simulink model "heaveCompMichael_v04"  (R2022b)
settings: Solver=VariableStepAuto  StartTime=0.0  StopTime=20  RelTol=1e-3
model workspace (MATLAB code in the model file):
  | %fluid data
  | rho = 875;
  | %valve config
  | P_r = 70e5;
  | Cd = 0.7;
  | Q_r = 200/6e4;
  | AdMax = Q_r/Cd/sqrt(2/rho*P_r/2);
  | 
  | g = 9.81;                   %gravity
  | zw = 0.8;                   %wave amplitude
  | tw = 10;                    %total wave period
  | ig = 46;                    %gear ratio gearbox
  | m = 9000;                   %mass of payload
  | mueq = 0.15;                %friction coeffisient
  | dd = 0.45;                  %diameter drum
  | nyv = 0.92;                 %volumetric effissiency
  | rd = dd/2;                  %radius drum
  | omega0 = 5;                 %velosity in friction equation
  | omegap = 1500;              %velosity hpu pump
  | nsh = 3;
  | gearrationsh = nsh.*2;
libraries: fl_lib x40, nesl_utility x24, sh_lib x7, slpidlib x2
(part 2 of 2)

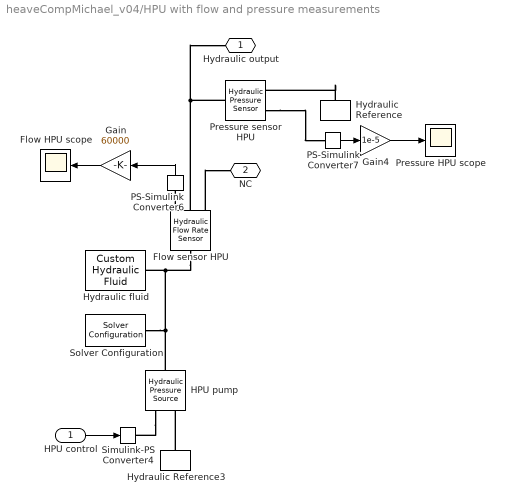
== system heaveCompMichael_v04/HPU with flow and pressure measurements ==
  HPU control : Inport
  Flow HPU scope : Scope
  Flow sensor HPU : fl_lib/Hydraulic/Hydraulic Sensors/Hydraulic Flow Rate Sensor
  Gain : Gain  Gain=60000
  Gain4 : Gain  Gain=1e-5
  HPU pump : fl_lib/Hydraulic/Hydraulic Sources/Hydraulic Pressure Source
      settings: InternalSimscapePortConfiguration="{\"Bottom\":[],\"Left\":[{\"id\":\"P\",\"label\":\"P\",\"type\":\"foundation.hydraulic.hydraulic\"}],\"Right\":[{\"id\":\"S\",\"label\":\"S\",\"type\":\"input\"},{\"id\":\"T\",\"label\":\"T\",\"type\":\"foundation.hydraulic.hydraulic\"}],\"Top\":[]}"
  Hydraulic Reference : fl_lib/Hydraulic/Hydraulic Elements/Hydraulic Reference
  Hydraulic Reference3 : fl_lib/Hydraulic/Hydraulic Elements/Hydraulic Reference
  Hydraulic fluid : fl_lib/Hydraulic/Hydraulic Utilities/Custom Hydraulic Fluid  density=875 kg/m^3  viscosity_kin=18e-6 m^2/s  bulk=0.8e9 Pa  alpha=0.005  range_error=2
      settings: InternalSimscapePortConfiguration="{\"Bottom\":[],\"Left\":[],\"Right\":[{\"id\":\"G\",\"label\":\"\",\"type\":\"foundation.hydraulic.hydraulic\"}],\"Top\":[]}"
  PS-Simulink Converter6 : nesl_utility/PS-Simulink Converter  PhysicalDomain=network_engine_domain  SubClassName=ps_output  LeftPortType=input  RightPortType=output  PseudoPeriodic=off  Frequencies=[]  VectorFormat=inherit  Unit=inherit  AffineConversion=off
  PS-Simulink Converter7 : nesl_utility/PS-Simulink Converter  PhysicalDomain=network_engine_domain  SubClassName=ps_output  LeftPortType=input  RightPortType=output  PseudoPeriodic=off  Frequencies=[]  VectorFormat=inherit  Unit=inherit  AffineConversion=off
  Pressure HPU scope : Scope
  Pressure sensor HPU : fl_lib/Hydraulic/Hydraulic Sensors/Hydraulic Pressure Sensor
  Simulink-PS Converter4 : nesl_utility/Simulink-PS Converter  PhysicalDomain=network_engine_domain  SubClassName=ps_input  LeftPortType=input  RightPortType=output  PseudoPeriodic=off  Frequencies=[]  NoiseDistribution=none  NoiseParameters=[]  Unit=1  AffineConversion=off  FilteringAndDerivatives=provide  SimscapeFilterOrder=1  InputFilterTimeConstant=0.001  UdotUserProvided=0
  Solver Configuration : nesl_utility/Solver Configuration  PhysicalDomain=network_engine_domain  SubClassName=solver  LeftPortType=input  RightPortType=generic  Tones=[]  Harmonics=[]  SimulateNoise=off  Profile=off  UseLocalSampling=off  EnableSwitchedLinearOptims=on  FrequencyDomain=off  UseCCode=off  RelTol=0.001  AbsTol=1e-06  MinStep=1e-09  ToWorkspace=off  RevertToSquareIcSolve=off  NumHomotopyIterations=100  PhasorMode=off  PhasorModeNumHarmonics=1  ConsistencySolver=NEWTON_FTOL  IndexReductionMethod=DerivativeReplacement  DoDC=off  ResidualTolerance=1e-09  ConsistencyTolSource=GLOBAL  ConsistencyAbsTol=0.001  ConsistencyRelTol=0.001  ConsistencyTolFactor=0.001  UseLocalSolver=off  LocalSolverChoice=NE_BACKWARD_EULER_ADVANCER  ResolveIndetEquations=on  FunctionEvalNumThread=1  LocalSolverSampleTime=0.001  DoFixedCost=off  MaxNonlinIter=3  MaxModeIter=2  ComputeImpulses=off  ImpulseIterations=2  LinearAlgebra=auto  LinearAlgebraNumThread=0  EquationFormulation=NE_TIME_EF  DelaysMemoryBudget=1024  AutomaticFiltering=on  FilteringTimeConstant=0.001  PartitionStorageMethod=AS_NEEDED  PartitionMemoryBudget=1024  PartitionMethod=ROBUST
  Hydraulic output : PMIOPort  Side=Right
  NC : PMIOPort  Port=2  Side=Right
  wires:
  PS-Simulink Converter6/1 -> Gain/1
  PS-Simulink Converter7/1 -> Gain4/1
  HPU control/1 -> Simulink-PS Converter4/1
  Gain/1 -> Flow HPU scope/1
  Gain4/1 -> Pressure HPU scope/1
  connections:
  HPU pump/LConn1 -- Solver Configuration/RConn1 -- Flow sensor HPU/LConn1 -- Hydraulic fluid/RConn1
  Hydraulic Reference3/LConn1 -- HPU pump/RConn2
  HPU pump/RConn1 -- Simulink-PS Converter4/RConn1
  Pressure sensor HPU/RConn2 -- PS-Simulink Converter7/LConn1
  Flow sensor HPU/RConn1 -- PS-Simulink Converter6/LConn1
  Flow sensor HPU/RConn2 -- Pressure sensor HPU/LConn1 -- Hydraulic output/RConn1
  Flow sensor HPU/RConn3 -- NC/RConn1
  Hydraulic Reference/LConn1 -- Pressure sensor HPU/RConn1

== matlab function heaveCompMichael_v04/MATLAB Function1 ==
  data: omega_m input; Mm output
function Mm = omega_m2Mm(omega_m)

n_sh = 3; % -
i_g = 46; % -
m_pl = 9000; % kg
d_D = 0.45; % m
mu_eq = 0.15; % -
omega_0 = 5; % rad/s
g = 9.81; % m/(s*s)

Mm = (m_pl*g*d_D)/(2*n_sh*2*i_g) * (1 + mu_eq * tanh(omega_m/omega_0));

== matlab function heaveCompMichael_v04/Brake valve control ==
  data: pressure input; u output
function u = fcn(pressure)

p_cr = 20; % bar
dp_fo = 10; % bar, delta p_fully_open

u = (pressure-p_cr)/dp_fo;

if(u >= 1)
    u = 1;
elseif(u < 0)
    u = 0;
end

== matlab function heaveCompMichael_v04/MATLAB Function2 ==
  data: t input; zp output; zp_dot output
function [zp, zp_dot]  = z_height(t)

z_w = 0.8; % m
T_w = 10; % s

zp = z_w * sin((2*pi*t)/T_w);
zp_dot = (2*z_w*pi*cos((2*pi*t)/T_w))/T_w;

== matlab function heaveCompMichael_v04/MATLAB Function ==
  data: u input; p output
function p = variable_pressure(u)

if(u > 0)
    p = 225e5; % Pa
else
    p = 40e5; % Pa
end

== matlab function heaveCompMichael_v04/MATLAB Function3 ==
  data: zp_dot input; u output; n output
function [u, n] = fcn(zp_dot)

dd = 0.45;
rho = 875; % kg/m^3

Dm = 28.1*10^-6; % m^3/rev
n = (zp_dot/(dd/2)) * 46  * 6 *2*pi; % rev/s

Q = (Dm*n);

Cd = 0.7;
Admax = (3.7646e-5)*2; % m^2

u = Q/(Cd*Admax * sqrt(2/rho*35e5));

== matlab function heaveCompMichael_v04/MATLAB Function4 ==
  data: t input; zp_ref output; zp_dot_ref output
function [zp_ref, zp_dot_ref]  = z_height(t)

z_w = 0.8; % m
T_w = 10; % s

zp_ref = z_w * sin((2*pi*t)/T_w);
zp_dot_ref = (2*z_w*pi*cos((2*pi*t)/T_w))/T_w;

== matlab function heaveCompMichael_v04/Variable pressure function ==
  data: u input; s output
function s = vp(u)

if(u < 0)
    s = 225e5;
else
    s = 225e5;
end

== matlab function heaveCompMichael_v04/MATLAB Function7 ==
  data: t input; omega_m input; Mm output
function Mm = motor_moment(t, omega_m)

n_sh = 3; % shieves
i_g = 46; % gearbox ratio
m_pl = 9000; % kg
d_D = 0.45; % m
mu_eq = 0.15; % -
omega_0 = 5; % rad/s
g = 9.81; % m/(s^2)

if(t < 10^-3)
    omega_m = 0;
end

Mm = ((m_pl*g*d_D)/(2*n_sh*2*i_g) * (1 + mu_eq * tanh(omega_m/omega_0)));

== matlab function heaveCompMichael_v04/MATLAB Function8 ==
  data: zp_dot input; u output; n output; Q output
function [u, n, Q] = fcn(zp_dot)

dd = 0.45;
rho = 875; % kg/m^3

Dm = 28.1*10^-6; % m^3/rev
n = (zp_dot/(dd/2)) * 46  * 6 / (2*pi); % rev/s

Q = (Dm*n);

Cd = 0.7;
Admax = (3.7646e-5); % m^2

u = Q/(Cd*Admax * sqrt(2/rho*35e5));

% m/s
